simulink model "pmsm_torque_estimator_wrapper"  (R2026a)
settings: Solver=FixedStepDiscrete  FixedStep=5e-5
libraries: mcbpmsmnonlinearlib x1
settings Model: Creator=hzldx  LastModifiedBy=hzldx
settings RTWCC: SystemTargetFile=ert.tlc  GenCodeOnly=on  GenerateMakefile=off  Description=Embedded Coder

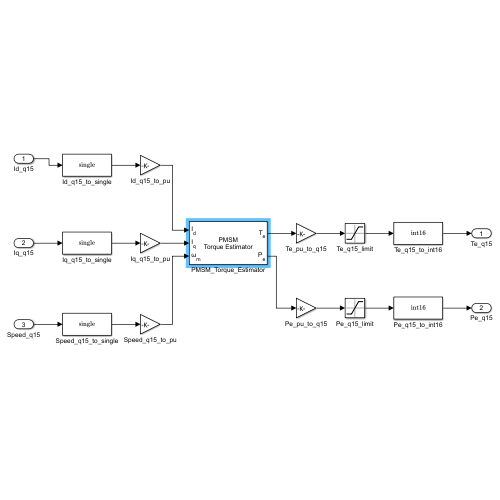
[thumbnail: Simulink's stored preview of the top-level diagram]
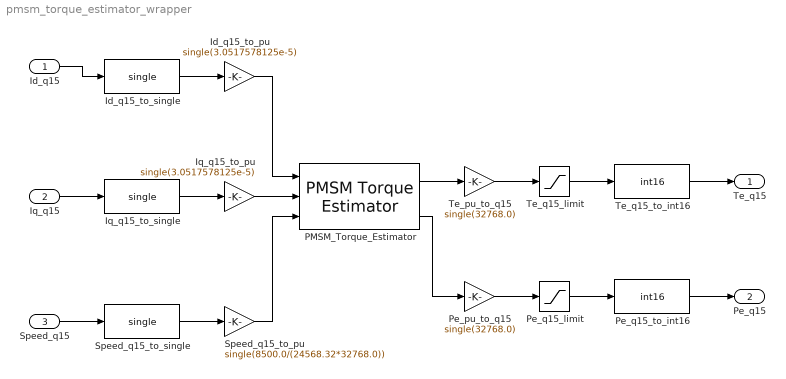
== system pmsm_torque_estimator_wrapper ==
  Id_q15 : Inport  OutDataTypeStr=int16
  Iq_q15 : Inport  Port=2  OutDataTypeStr=int16
  Speed_q15 : Inport  Port=3  OutDataTypeStr=int16
  Id_q15_to_pu : Gain  Gain=single(3.0517578125e-5)  OutDataTypeStr=single
  Id_q15_to_single : DataTypeConversion  OutDataTypeStr=single  SaturateOnIntegerOverflow=off  RndMeth=Floor
  Iq_q15_to_pu : Gain  Gain=single(3.0517578125e-5)  OutDataTypeStr=single
  Iq_q15_to_single : DataTypeConversion  OutDataTypeStr=single  SaturateOnIntegerOverflow=off  RndMeth=Floor
  PMSM_Torque_Estimator : mcbpmsmnonlinearlib/PMSM Torque Estimator  polePairs=4  nonLinearityChoice=Linear model with lumped parameters  Ld=0.0012  Lq=0.0023  FluxPM=0.032390572606  idVec=[-40, -20, 0, 20]  iqVec=[-40, -20, 0, 20, 40]  LdTable=0.2e-3 * ones(4, 5)  LqTable=0.2e-3 * ones(4, 5)  FluxPMTable=6.4e-3 * ones(4, 5)  FluxDTable=[-1.6,-1.6,-1.6,-1.6,-1.6;2.4,2.4,2.4,2.4,2.4;6.4,6.4,6.4,6.4,6.4;10.4,10.4,10.4,10.4,10.4]*1e-3  FluxQTable=[-8,-4,0,4,8;-8,-4,0,4,8;-8,-4,0,4,8;-8,-4,0,4,8]*1e-3  Units=Per-Unit (PU)  V_base=1000/sqrt(3)  I_base=50  N_base=24568.32  T_base=9.7172  P_base=43301.2702  scaledTables=on
      settings: LibrarySourceBlock=mcblib/Controls/Control Reference/PMSM Torque Estimator
  Pe_pu_to_q15 : Gain  Gain=single(32768.0)  OutDataTypeStr=single
  Pe_q15_limit : Saturate  UpperLimit=32767.0  LowerLimit=-32768.0
  Pe_q15_to_int16 : DataTypeConversion  OutDataTypeStr=int16
  Speed_q15_to_pu : Gain  Gain=single(8500.0/(24568.32*32768.0))  OutDataTypeStr=single
  Speed_q15_to_single : DataTypeConversion  OutDataTypeStr=single  SaturateOnIntegerOverflow=off  RndMeth=Floor
  Te_pu_to_q15 : Gain  Gain=single(32768.0)  OutDataTypeStr=single
  Te_q15_limit : Saturate  UpperLimit=32767.0  LowerLimit=-32768.0
  Te_q15_to_int16 : DataTypeConversion  OutDataTypeStr=int16
  Te_q15 : Outport  OutDataTypeStr=int16
  Pe_q15 : Outport  Port=2  OutDataTypeStr=int16
  wires:
  Id_q15/1 -> Id_q15_to_single/1
  Id_q15_to_single/1 -> Id_q15_to_pu/1
  Id_q15_to_pu/1 -> PMSM_Torque_Estimator/1
  Iq_q15/1 -> Iq_q15_to_single/1
  Iq_q15_to_single/1 -> Iq_q15_to_pu/1
  Iq_q15_to_pu/1 -> PMSM_Torque_Estimator/2
  Speed_q15/1 -> Speed_q15_to_single/1
  Speed_q15_to_single/1 -> Speed_q15_to_pu/1
  Speed_q15_to_pu/1 -> PMSM_Torque_Estimator/3
  PMSM_Torque_Estimator/1 -> Te_pu_to_q15/1
  Te_pu_to_q15/1 -> Te_q15_limit/1
  Te_q15_limit/1 -> Te_q15_to_int16/1
  Te_q15_to_int16/1 -> Te_q15/1
  PMSM_Torque_Estimator/2 -> Pe_pu_to_q15/1
  Pe_pu_to_q15/1 -> Pe_q15_limit/1
  Pe_q15_limit/1 -> Pe_q15_to_int16/1
  Pe_q15_to_int16/1 -> Pe_q15/1
